simulink model "OswaldE_Proj2_Sim"  (R2024b)
settings: Solver=ode45  StartTime=0.0  StopTime=300  RelTol=1e-3  AbsTol=1e-6
values from neighbouring files (symbols this model uses):
  g0 = 32.17    [OswaldE_Proj2_Code.m]
  gamma_0 = 0    [OswaldE_Proj2_Code.m]
  h_0 = 20000    [OswaldE_Proj2_Code.m]
  K_f = 4*10^-6    (= 4e-06)    [OswaldE_Proj2_Code.m]
  K_L_max = 2.6    [OswaldE_Proj2_Code.m]
  K_mu_p = 0.075    [OswaldE_Proj2_Code.m]
  KL_i = 0.01    [OswaldE_Proj2_Code.m]
  KL_p = 0.5    [OswaldE_Proj2_Code.m]
  KT_i = 0.002    [OswaldE_Proj2_Code.m]
  KT_p = 0.08    [OswaldE_Proj2_Code.m]
  lat_0 = 33.2098 * pi/180    (= 0.579620353929)    [OswaldE_Proj2_Code.m]
  long_0 = -87.5692 * pi/180    (= -1.52837086334)    [OswaldE_Proj2_Code.m]
  mu_max = 30    [OswaldE_Proj2_Code.m]
  omega_L = 2.5    [OswaldE_Proj2_Code.m]
  omega_mu = 1    [OswaldE_Proj2_Code.m]
  omega_t = 2    [OswaldE_Proj2_Code.m]
  sigma_0 = 0    [OswaldE_Proj2_Code.m]
  T_max = 72000    [OswaldE_Proj2_Code.m]
  v_bn_0 = 600    [OswaldE_Proj2_Code.m]
  weight_0 = 200000    [OswaldE_Proj2_Code.m]
libraries: simulink_extras x8, simulink x2
settings Model: Creator=jdlarson1  LastModifiedBy=ethan
settings SolverCC: AlgebraicLoopSolver=TrustRegion
settings DataIOCC: SaveFormat=Array  SignalLoggingSaveFormat=ModelDataLogs  ReturnWorkspaceOutputs=off
settings OptimizationCC: BlockReduction=off  BooleanDataType=off  ReuseModelBlockBuffer=off
settings DebuggingCC: SaveWithParameterizedLinksMsg=none  UnderspecifiedInitializationDetection=Classic  MergeDetectMultiDrivingBlocksExec=none  SignalResolutionControl=TryResolveAllWithWarning  MultiTaskDSMMsg=warning  MultiTaskCondExecSysMsg=none  UnconnectedInputMsg=warning  UnconnectedOutputMsg=warning  UnconnectedLineMsg=warning
settings HardwareCC: TargetUnknown=on
settings ModelReferenceCC: EnableRefExpFcnMdlSchedulingChecks=on  PropagateSignalLabelsOutOfModel=off
settings RTWCC: GPUComputeCapability=3.5  DLArmComputeVersion=19.05
settings GRTTargetCC: CombineOutputUpdateFcns=off  GRTInterface=on

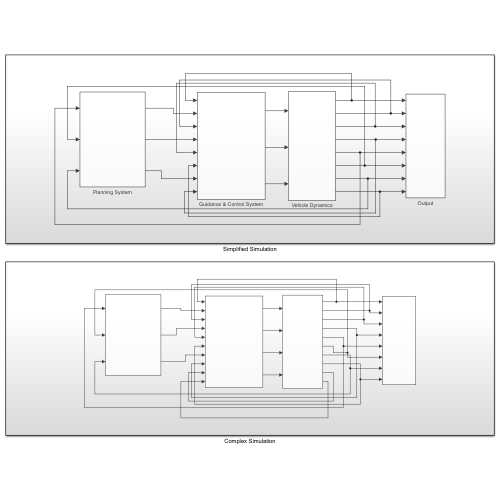
[thumbnail: Simulink's stored preview of the top-level diagram]
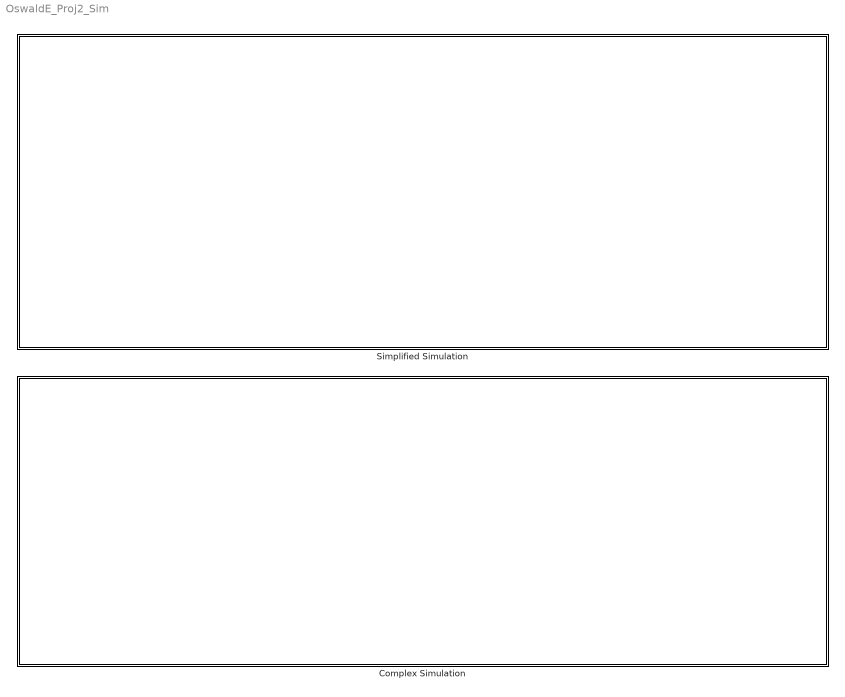
== system OswaldE_Proj2_Sim ==
  Complex Simulation : Subsystem
  Simplified Simulation : Subsystem

== system OswaldE_Proj2_Sim/Complex Simulation ==
  Guidance & Control System1 : Subsystem
  Output1 : Subsystem
  Planning System1 : Subsystem
  Vehicle Dynamics1 : Subsystem
  wires:
  Vehicle Dynamics1/2(" groundspeed ") -> Output1/2(groundspeed), Guidance & Control System1/3(groundspeed)
  Planning System1/2(flight-path_com) -> Guidance & Control System1/4(flight-path_com)
  Vehicle Dynamics1/3(" flight-path ") -> Output1/3(flight-path), Guidance & Control System1/5(flight-path)
  Vehicle Dynamics1/4(" heading ") -> Guidance & Control System1/8(heading), Output1/4(heading)
  Vehicle Dynamics1/7(altitude) -> Planning System1/3(altitude), Output1/7(altitude)
  Vehicle Dynamics1/10(rho) -> Guidance & Control System1/10(rho)
  Guidance & Control System1/3(bank) -> Vehicle Dynamics1/3(bank)
  Vehicle Dynamics1/8(airspeed) -> Guidance & Control System1/6(airspeed), Output1/8(airspeed)
  Vehicle Dynamics1/5(latitude) -> Planning System1/1(latitude), Output1/5(latitude)
  Planning System1/3(heading_com) -> Guidance & Control System1/7(heading_com)
  Vehicle Dynamics1/6(longitude) -> Output1/6(longitude), Planning System1/2(longitude)
  Guidance & Control System1/4(alpha) -> Vehicle Dynamics1/4(alpha)
  Vehicle Dynamics1/1(" mass") -> Guidance & Control System1/1(mass), Output1/1(mass)
  Guidance & Control System1/1(thrust) -> Vehicle Dynamics1/1("thrust ")
  Guidance & Control System1/2(lift) -> Vehicle Dynamics1/2("lift ")
  Planning System1/1(groundspeed_com) -> Guidance & Control System1/2(groundspeed_com)
  Vehicle Dynamics1/9(g) -> Guidance & Control System1/9(g)

== system OswaldE_Proj2_Sim/Simplified Simulation ==
  Guidance & Control System : Subsystem
  Output : Subsystem
  Planning System : Subsystem
  Vehicle Dynamics : Subsystem
  wires:
  Vehicle Dynamics/2(" groundspeed ") -> Guidance & Control System/3(groundspeed), Output/2(groundspeed)
  Vehicle Dynamics/5(latitude) -> Planning System/1(latitude), Output/5(latitude)
  Vehicle Dynamics/7(altitude) -> Planning System/3(altitude), Output/7(altitude)
  Vehicle Dynamics/3(" flight-path ") -> Guidance & Control System/5(flight-path), Output/3(flight-path)
  Planning System/1(groundspeed_com) -> Guidance & Control System/2(groundspeed_com)
  Guidance & Control System/2(lift) -> Vehicle Dynamics/2("lift ")
  Guidance & Control System/1(thrust) -> Vehicle Dynamics/1("thrust ")
  Vehicle Dynamics/1(" mass") -> Output/1(mass), Guidance & Control System/1(mass)
  Vehicle Dynamics/4(" heading ") -> Guidance & Control System/8(heading), Output/4(heading)
  Guidance & Control System/3(bank) -> Vehicle Dynamics/3(bank)
  Vehicle Dynamics/8(airspeed) -> Guidance & Control System/6(airspeed), Output/8(airspeed)
  Vehicle Dynamics/6(longitude) -> Planning System/2(longitude), Output/6(longitude)
  Planning System/3(heading_com) -> Guidance & Control System/7(heading_com)
  Planning System/2(flight-path_com) -> Guidance & Control System/4(flight-path_com)

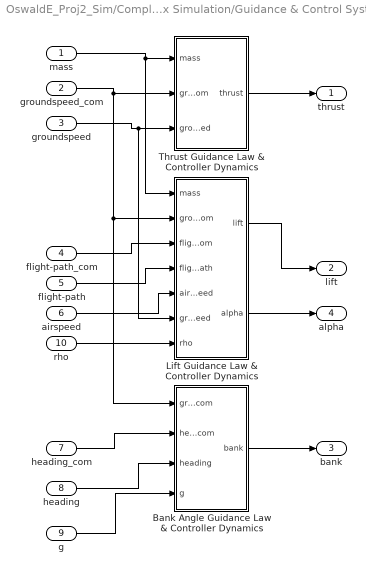
== system OswaldE_Proj2_Sim/Complex Simulation/Guidance & Control System1 ==
  mass : Inport
  groundspeed_com : Inport  Port=2
  groundspeed : Inport  Port=3
  flight-path_com : Inport  Port=4
  flight-path : Inport  Port=5
  airspeed : Inport  Port=6
  heading_com : Inport  Port=7
  heading : Inport  Port=8
  g : Inport  Port=9
  rho : Inport  Port=10
  Bank Angle Guidance Law & Controller Dynamics : Subsystem
  Lift Guidance Law & Controller Dynamics : Subsystem
  Thrust Guidance Law & Controller Dynamics : Subsystem
  thrust : Outport
  lift : Outport  Port=2
  bank : Outport  Port=3
  alpha : Outport  Port=4
  wires:
  mass/1 -> Lift Guidance Law & Controller Dynamics/1(mass), Thrust Guidance Law & Controller Dynamics/1(mass)
  heading_com/1 -> Bank Angle Guidance Law & Controller Dynamics/2(heading_com)
  groundspeed/1 -> Thrust Guidance Law & Controller Dynamics/3(groundspeed), Lift Guidance Law & Controller Dynamics/6(groundspeed)
  groundspeed_com/1 -> Bank Angle Guidance Law & Controller Dynamics/1(groundspeed_com), Lift Guidance Law & Controller Dynamics/2(groundspeed_com), Thrust Guidance Law & Controller Dynamics/2(groundspeed_com)
  heading/1 -> Bank Angle Guidance Law & Controller Dynamics/3(heading)
  flight-path/1 -> Lift Guidance Law & Controller Dynamics/4(flight_path)
  airspeed/1 -> Lift Guidance Law & Controller Dynamics/5(airspeed)
  Thrust Guidance Law & Controller Dynamics/1(thrust) -> thrust/1
  Lift Guidance Law & Controller Dynamics/1(lift) -> lift/1
  Bank Angle Guidance Law & Controller Dynamics/1(bank) -> bank/1
  flight-path_com/1 -> Lift Guidance Law & Controller Dynamics/3(flight_path_com)
  g/1 -> Bank Angle Guidance Law & Controller Dynamics/4(g)
  Lift Guidance Law & Controller Dynamics/2(alpha) -> alpha/1
  rho/1 -> Lift Guidance Law & Controller Dynamics/7(rho)

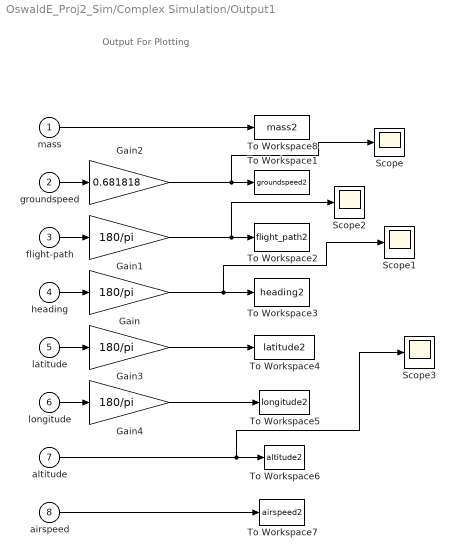
== system OswaldE_Proj2_Sim/Complex Simulation/Output1 ==
  note: Output For Plotting
  mass : Inport
  groundspeed : Inport  Port=2
  flight-path : Inport  Port=3
  heading : Inport  Port=4
  latitude : Inport  Port=5
  longitude : Inport  Port=6
  altitude : Inport  Port=7
  airspeed : Inport  Port=8
  Gain{,1,3..4} (4 alike) : Gain  Gain=180/pi
  Gain2 : Gain  Gain=0.681818
  Scope{,1..3} (4 alike) : Scope
  To Workspace1 : ToWorkspace  VariableName=groundspeed2
  To Workspace2 : ToWorkspace  VariableName=flight_path2
  To Workspace3 : ToWorkspace  VariableName=heading2
  To Workspace4 : ToWorkspace  VariableName=latitude2
  To Workspace5 : ToWorkspace  VariableName=longitude2
  To Workspace6 : ToWorkspace  VariableName=altitude2
  To Workspace7 : ToWorkspace  VariableName=airspeed2
  To Workspace8 : ToWorkspace  VariableName=mass2
  wires:
  latitude/1 -> Gain3/1
  groundspeed/1 -> Gain2/1
  flight-path/1 -> Gain1/1
  heading/1 -> Gain/1
  longitude/1 -> Gain4/1
  altitude/1 -> Scope3/1, To Workspace6/1
  Gain2/1 -> Scope/1, To Workspace1/1
  Gain1/1 -> Scope2/1, To Workspace2/1
  Gain/1 -> Scope1/1, To Workspace3/1
  airspeed/1 -> To Workspace7/1
  mass/1 -> To Workspace8/1
  Gain3/1 -> To Workspace4/1
  Gain4/1 -> To Workspace5/1

== system OswaldE_Proj2_Sim/Complex Simulation/Planning System1 ==
  latitude : Inport
  longitude : Inport  Port=2
  altitude : Inport  Port=3
  CD1 : Gain  Gain=180/pi  SaturateOnIntegerOverflow=on
  CD7 : Gain  Gain=180/pi  SaturateOnIntegerOverflow=on
  CD8 : Gain  Gain=0.681818  SaturateOnIntegerOverflow=on
  Command System : MATLAB Function  TreatAsAtomicUnit=on
  To Workspace10 : ToWorkspace  VariableName=heading_com2
  To Workspace5 : ToWorkspace  VariableName=groundspeed_com2
  To Workspace7 : ToWorkspace  VariableName=flight_path_com2
  groundspeed_com : Outport
  flight-path_com : Outport  Port=2
  heading_com : Outport  Port=3
  wires:
  latitude/1 -> Command System/1(latitude)
  longitude/1 -> Command System/2(longitude)
  altitude/1 -> Command System/3(altitude)
  Command System/1(groundspeed_com) -> CD8/1, groundspeed_com/1
  Command System/2(flight_path_com) -> CD7/1, flight-path_com/1
  Command System/3(heading_com) -> CD1/1, heading_com/1
  CD8/1 -> To Workspace5/1
  CD7/1 -> To Workspace7/1
  CD1/1 -> To Workspace10/1

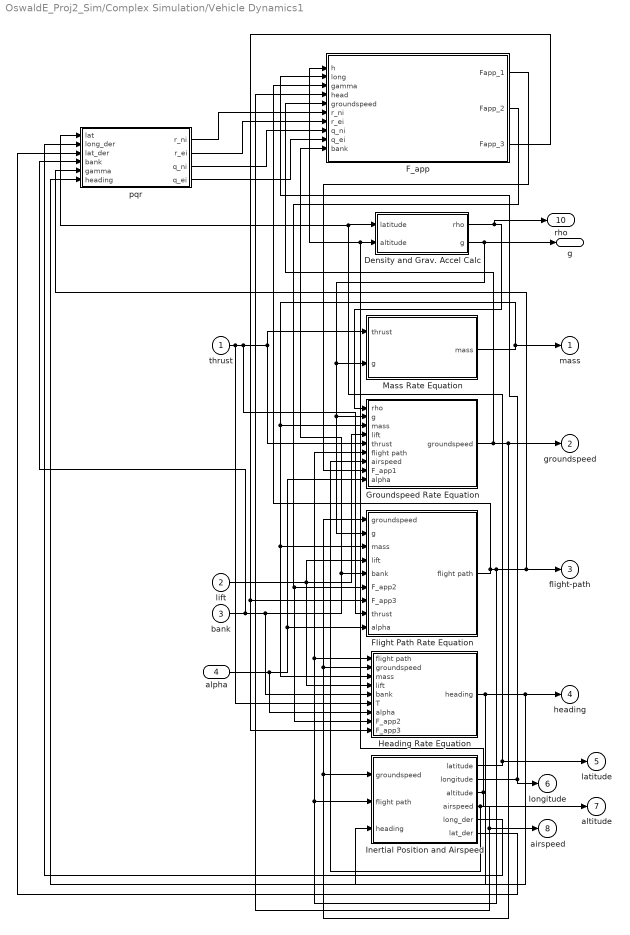
== system OswaldE_Proj2_Sim/Complex Simulation/Vehicle Dynamics1 ==
  "thrust " : Inport
  "lift " : Inport  Port=2
  bank : Inport  Port=3
  alpha : Inport  Port=4
  Density and Grav. Accel Calc : Subsystem
  F_app : Subsystem
  Flight Path Rate Equation : Subsystem
  Groundspeed Rate Equation : Subsystem
  Heading Rate Equation : Subsystem
  Inertial Position and Airspeed : Subsystem
  Mass Rate Equation : Subsystem
  pqr : Subsystem
  " mass" : Outport
  " groundspeed " : Outport  Port=2
  " flight-path " : Outport  Port=3
  " heading " : Outport  Port=4
  latitude : Outport  Port=5
  longitude : Outport  Port=6
  altitude : Outport  Port=7
  airspeed : Outport  Port=8
  g : Outport  Port=9
  rho : Outport  Port=10
  wires:
  bank/1 -> pqr/4(bank), F_app/10(bank), Flight Path Rate Equation/5(bank), Heading Rate Equation/5(bank)
  "lift "/1 -> Heading Rate Equation/4("lift "), Flight Path Rate Equation/4("lift "), Groundspeed Rate Equation/4(lift)
  "thrust "/1 -> Heading Rate Equation/6(T), Flight Path Rate Equation/8(thrust), Groundspeed Rate Equation/5(thrust), Mass Rate Equation/1(thrust)
  Heading Rate Equation/1(heading) -> Inertial Position and Airspeed/3(heading), " heading "/1, pqr/6(heading)
  Flight Path Rate Equation/1(flight path) -> F_app/3(gamma), Groundspeed Rate Equation/6(flight path), Heading Rate Equation/1(flight path), Inertial Position and Airspeed/2("flight path "), pqr/5(gamma), " flight-path "/1
  Groundspeed Rate Equation/1(groundspeed) -> F_app/5(groundspeed), Flight Path Rate Equation/1(groundspeed), Heading Rate Equation/2(groundspeed), Inertial Position and Airspeed/1(groundspeed), " groundspeed "/1
  Inertial Position and Airspeed/2(longitude) -> longitude/1, F_app/2(long)
  Inertial Position and Airspeed/4(airspeed) -> F_app/4(head), airspeed/1, Groundspeed Rate Equation/7(airspeed)
  Inertial Position and Airspeed/1(latitude) -> pqr/1(lat), Density and Grav. Accel Calc/1(latitude), latitude/1
  Inertial Position and Airspeed/3(altitude) -> altitude/1, F_app/1(h), Density and Grav. Accel Calc/2(altitude)
  Mass Rate Equation/1("mass ") -> " mass"/1, Heading Rate Equation/3(mass), Flight Path Rate Equation/3(mass), Groundspeed Rate Equation/3(mass)
  Density and Grav. Accel Calc/1(rho) -> rho/1, Groundspeed Rate Equation/1(rho)
  Density and Grav. Accel Calc/2(g) -> g/1, Flight Path Rate Equation/2(g), Groundspeed Rate Equation/2(g), Mass Rate Equation/2(g)
  pqr/1(r_ni) -> F_app/6(r_ni)
  pqr/2(r_ei) -> F_app/7(r_ei)
  pqr/3(q_ni) -> F_app/8(q_ni)
  pqr/4(q_ei) -> F_app/9(q_ei)
  Inertial Position and Airspeed/5(long_der) -> pqr/2(long_der)
  Inertial Position and Airspeed/6(lat_der) -> pqr/3(lat_der)
  F_app/1(Fapp_1) -> Groundspeed Rate Equation/8(F_app1)
  F_app/2(Fapp_2) -> Heading Rate Equation/8(F_app2), Flight Path Rate Equation/6(F_app2)
  F_app/3(Fapp_3) -> Heading Rate Equation/9(F_app3), Flight Path Rate Equation/7(F_app3)
  alpha/1 -> Heading Rate Equation/7(alpha), Groundspeed Rate Equation/9(alpha), Flight Path Rate Equation/9(alpha)

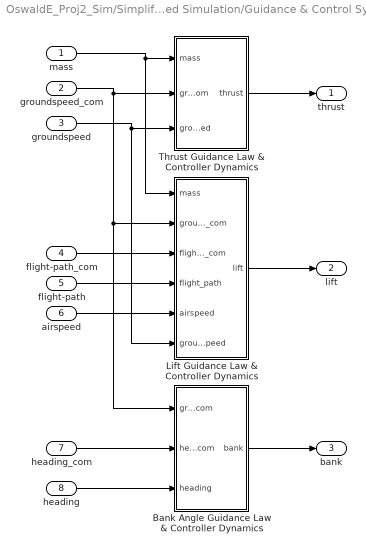
== system OswaldE_Proj2_Sim/Simplified Simulation/Guidance & Control System ==
  mass : Inport
  groundspeed_com : Inport  Port=2
  groundspeed : Inport  Port=3
  flight-path_com : Inport  Port=4
  flight-path : Inport  Port=5
  airspeed : Inport  Port=6
  heading_com : Inport  Port=7
  heading : Inport  Port=8
  Bank Angle Guidance Law & Controller Dynamics : Subsystem
  Lift Guidance Law & Controller Dynamics : Subsystem
  Thrust Guidance Law & Controller Dynamics : Subsystem
  thrust : Outport
  lift : Outport  Port=2
  bank : Outport  Port=3
  wires:
  mass/1 -> Lift Guidance Law & Controller Dynamics/1(mass), Thrust Guidance Law & Controller Dynamics/1(mass)
  heading_com/1 -> Bank Angle Guidance Law & Controller Dynamics/2(heading_com)
  groundspeed/1 -> Thrust Guidance Law & Controller Dynamics/3(groundspeed), Lift Guidance Law & Controller Dynamics/6(groundspeed)
  groundspeed_com/1 -> Lift Guidance Law & Controller Dynamics/2(groundspeed_com), Bank Angle Guidance Law & Controller Dynamics/1(groundspeed_com), Thrust Guidance Law & Controller Dynamics/2(groundspeed_com)
  heading/1 -> Bank Angle Guidance Law & Controller Dynamics/3(heading)
  flight-path/1 -> Lift Guidance Law & Controller Dynamics/4(flight_path)
  airspeed/1 -> Lift Guidance Law & Controller Dynamics/5(airspeed)
  Thrust Guidance Law & Controller Dynamics/1(thrust) -> thrust/1
  Lift Guidance Law & Controller Dynamics/1(lift) -> lift/1
  Bank Angle Guidance Law & Controller Dynamics/1(bank) -> bank/1
  flight-path_com/1 -> Lift Guidance Law & Controller Dynamics/3(flight_path_com)

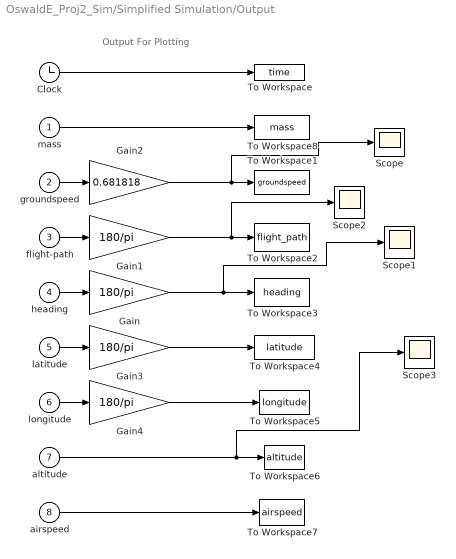
== system OswaldE_Proj2_Sim/Simplified Simulation/Output ==
  note: Output For Plotting
  mass : Inport
  groundspeed : Inport  Port=2
  flight-path : Inport  Port=3
  heading : Inport  Port=4
  latitude : Inport  Port=5
  longitude : Inport  Port=6
  altitude : Inport  Port=7
  airspeed : Inport  Port=8
  Clock : Clock
  Gain{,1,3..4} (4 alike) : Gain  Gain=180/pi
  Gain2 : Gain  Gain=0.681818
  Scope{,1..3} (4 alike) : Scope
  To Workspace : ToWorkspace  VariableName=time
  To Workspace1 : ToWorkspace  VariableName=groundspeed
  To Workspace2 : ToWorkspace  VariableName=flight_path
  To Workspace3 : ToWorkspace  VariableName=heading
  To Workspace4 : ToWorkspace  VariableName=latitude
  To Workspace5 : ToWorkspace  VariableName=longitude
  To Workspace6 : ToWorkspace  VariableName=altitude
  To Workspace7 : ToWorkspace  VariableName=airspeed
  To Workspace8 : ToWorkspace  VariableName=mass
  wires:
  Clock/1 -> To Workspace/1
  latitude/1 -> Gain3/1
  groundspeed/1 -> Gain2/1
  flight-path/1 -> Gain1/1
  heading/1 -> Gain/1
  longitude/1 -> Gain4/1
  altitude/1 -> Scope3/1, To Workspace6/1
  Gain2/1 -> Scope/1, To Workspace1/1
  Gain1/1 -> Scope2/1, To Workspace2/1
  Gain/1 -> Scope1/1, To Workspace3/1
  airspeed/1 -> To Workspace7/1
  mass/1 -> To Workspace8/1
  Gain3/1 -> To Workspace4/1
  Gain4/1 -> To Workspace5/1

== system OswaldE_Proj2_Sim/Simplified Simulation/Planning System ==
  latitude : Inport
  longitude : Inport  Port=2
  altitude : Inport  Port=3
  CD1 : Gain  Gain=180/pi  SaturateOnIntegerOverflow=on
  CD7 : Gain  Gain=180/pi  SaturateOnIntegerOverflow=on
  CD8 : Gain  Gain=0.681818  SaturateOnIntegerOverflow=on
  Command System : MATLAB Function  TreatAsAtomicUnit=on
  To Workspace10 : ToWorkspace  VariableName=heading_com
  To Workspace5 : ToWorkspace  VariableName=groundspeed_com
  To Workspace7 : ToWorkspace  VariableName=flight_path_com
  groundspeed_com : Outport
  flight-path_com : Outport  Port=2
  heading_com : Outport  Port=3
  wires:
  latitude/1 -> Command System/1(latitude)
  longitude/1 -> Command System/2(longitude)
  altitude/1 -> Command System/3(altitude)
  Command System/1(groundspeed_com) -> CD8/1, groundspeed_com/1
  Command System/2(flight_path_com) -> CD7/1, flight-path_com/1
  Command System/3(heading_com) -> CD1/1, heading_com/1
  CD8/1 -> To Workspace5/1
  CD7/1 -> To Workspace7/1
  CD1/1 -> To Workspace10/1

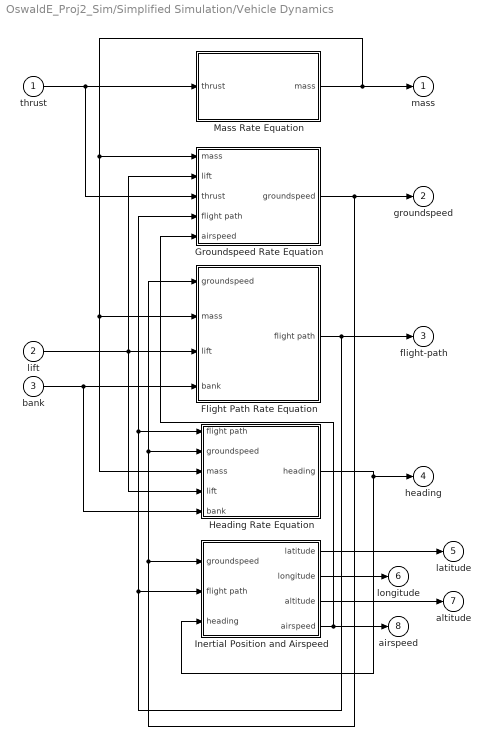
== system OswaldE_Proj2_Sim/Simplified Simulation/Vehicle Dynamics ==
  "thrust " : Inport
  "lift " : Inport  Port=2
  bank : Inport  Port=3
  Flight Path Rate Equation : Subsystem
  Groundspeed Rate Equation : Subsystem
  Heading Rate Equation : Subsystem
  Inertial Position and Airspeed : Subsystem
  Mass Rate Equation : Subsystem
  " mass" : Outport
  " groundspeed " : Outport  Port=2
  " flight-path " : Outport  Port=3
  " heading " : Outport  Port=4
  latitude : Outport  Port=5
  longitude : Outport  Port=6
  altitude : Outport  Port=7
  airspeed : Outport  Port=8
  wires:
  bank/1 -> Heading Rate Equation/5(bank), Flight Path Rate Equation/4(bank)
  "lift "/1 -> Heading Rate Equation/4("lift "), Flight Path Rate Equation/3("lift "), Groundspeed Rate Equation/2(lift)
  "thrust "/1 -> Groundspeed Rate Equation/3(thrust), Mass Rate Equation/1(thrust)
  Heading Rate Equation/1(heading) -> Inertial Position and Airspeed/3(heading), " heading "/1
  Flight Path Rate Equation/1(flight path) -> Groundspeed Rate Equation/4(flight path), Heading Rate Equation/1(flight path), Inertial Position and Airspeed/2("flight path "), " flight-path "/1
  Groundspeed Rate Equation/1(groundspeed) -> Flight Path Rate Equation/1(groundspeed), Heading Rate Equation/2(groundspeed), Inertial Position and Airspeed/1(groundspeed), " groundspeed "/1
  Inertial Position and Airspeed/2(longitude) -> longitude/1
  Inertial Position and Airspeed/4(airspeed) -> Groundspeed Rate Equation/5(airspeed), airspeed/1
  Inertial Position and Airspeed/1(latitude) -> latitude/1
  Inertial Position and Airspeed/3(altitude) -> altitude/1
  Mass Rate Equation/1("mass ") -> " mass"/1, Heading Rate Equation/3(mass), Flight Path Rate Equation/2(mass), Groundspeed Rate Equation/1(mass)

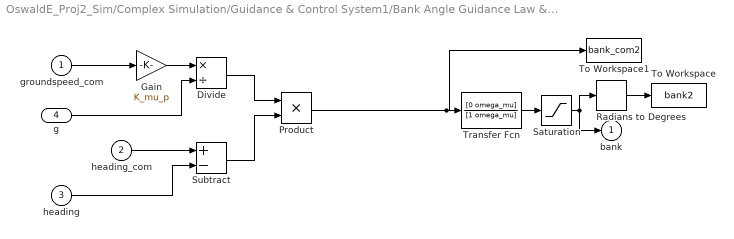
== system OswaldE_Proj2_Sim/Complex Simulation/Guidance & Control System1/Bank Angle Guidance Law & Controller Dynamics ==
  groundspeed_com : Inport
  heading_com : Inport  Port=2
  heading : Inport  Port=3
  g : Inport  Port=4
  Divide : Product  Inputs=*/
  Gain : Gain  Gain=K_mu_p
  Product : Product
  Radians to Degrees : simulink_extras/Transformations/Radians to Degrees
  Saturation : Saturate  UpperLimit=mu_max*pi/180  LowerLimit=-mu_max*pi/180
  Subtract : Sum  Inputs=+-
  To Workspace : ToWorkspace  VariableName=bank2
  To Workspace1 : ToWorkspace  VariableName=bank_com2
  Transfer Fcn : TransferFcn  Numerator=[0 omega_mu]  Denominator=[1 omega_mu]
  bank : Outport
  wires:
  groundspeed_com/1 -> Gain/1
  Gain/1 -> Divide/1
  g/1 -> Divide/2
  heading_com/1 -> Subtract/1
  heading/1 -> Subtract/2
  Divide/1 -> Product/1
  Subtract/1 -> Product/2
  Product/1 -> To Workspace1/1, Transfer Fcn/1
  Transfer Fcn/1 -> Saturation/1
  Saturation/1 -> bank/1, Radians to Degrees/1
  Radians to Degrees/1 -> To Workspace/1

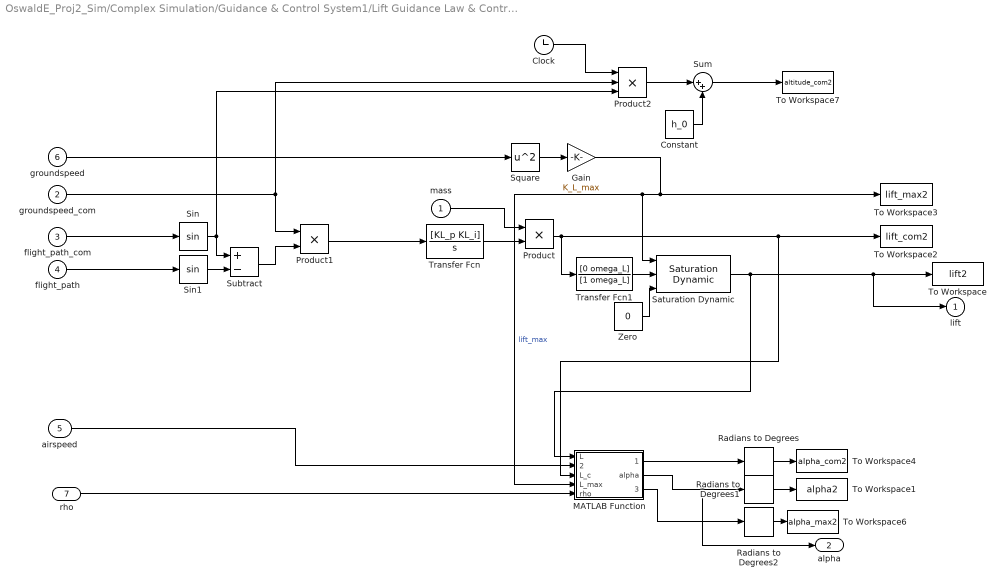
== system OswaldE_Proj2_Sim/Complex Simulation/Guidance & Control System1/Lift Guidance Law & Controller Dynamics ==
  mass : Inport
  groundspeed_com : Inport  Port=2
  flight_path_com : Inport  Port=3
  flight_path : Inport  Port=4
  airspeed : Inport  Port=5
  groundspeed : Inport  Port=6
  rho : Inport  Port=7
  Clock : Clock
  Constant : Constant  Value=h_0
  Gain : Gain  Gain=K_L_max
  MATLAB Function : MATLAB Function  TreatAsAtomicUnit=on
  Product : Product
  Product1 : Product
  Product2 : Product  Inputs=3
  Radians to Degrees : simulink_extras/Transformations/Radians to Degrees
  Radians to Degrees1 : simulink_extras/Transformations/Radians to Degrees
  Radians to Degrees2 : simulink_extras/Transformations/Radians to Degrees
  Saturation Dynamic : simulink/Discontinuities/Saturation Dynamic  OutMin=[]  OutMax=[]  OutDataTypeStr=Inherit: Same as second input  OutDataType=fixdt(1, 16)  OutScaling=2^-10  DoSatur=off
  Sin : Trigonometry
  Sin1 : Trigonometry
  Square : Math  Operator=square
  Subtract : Sum  Inputs=+-
  Sum : Sum  Inputs=|++
  To Workspace : ToWorkspace  VariableName=lift2
  To Workspace1 : ToWorkspace  VariableName=alpha2
  To Workspace2 : ToWorkspace  VariableName=lift_com2
  To Workspace3 : ToWorkspace  VariableName=lift_max2
  To Workspace4 : ToWorkspace  VariableName=alpha_com2
  To Workspace6 : ToWorkspace  VariableName=alpha_max2
  To Workspace7 : ToWorkspace  VariableName=altitude_com2
  Transfer Fcn : TransferFcn  Numerator=[KL_p KL_i]  Denominator=[1 0]
  Transfer Fcn1 : TransferFcn  Numerator=[0 omega_L]  Denominator=[1 omega_L]
  Zero : Constant  Value=0  OutDataTypeStr=Inherit: Inherit via back propagation
  lift : Outport
  alpha : Outport  Port=2
  wires:
  Transfer Fcn/1 -> Product/2
  mass/1 -> Product/1
  flight_path_com/1 -> Sin/1
  Sin/1 -> Subtract/1, Product2/3
  flight_path/1 -> Sin1/1
  Sin1/1 -> Subtract/2
  Subtract/1 -> Product1/2
  groundspeed_com/1 -> Product2/2, Product1/1
  Product1/1 -> Transfer Fcn/1
  Product/1 -> Transfer Fcn1/1, MATLAB Function/3(L_c), To Workspace2/1
  groundspeed/1 -> Square/1
  Square/1 -> Gain/1
  Gain/1 -> MATLAB Function/4(L_max), Saturation Dynamic/1, To Workspace3/1  "lift_max"
  airspeed/1 -> MATLAB Function/2(airspeed)
  MATLAB Function/2(alpha) -> Radians to Degrees1/1, alpha/1
  Transfer Fcn1/1 -> Saturation Dynamic/2
  Saturation Dynamic/1 -> MATLAB Function/1(L), lift/1, To Workspace/1
  Zero/1 -> Saturation Dynamic/3
  Clock/1 -> Product2/1
  Product2/1 -> Sum/1
  Constant/1 -> Sum/2
  Sum/1 -> To Workspace7/1
  rho/1 -> MATLAB Function/5(rho)
  Radians to Degrees/1 -> To Workspace4/1
  MATLAB Function/1(alpha_c) -> Radians to Degrees/1
  Radians to Degrees1/1 -> To Workspace1/1
  MATLAB Function/3(alpha_max) -> Radians to Degrees2/1
  Radians to Degrees2/1 -> To Workspace6/1

== system OswaldE_Proj2_Sim/Complex Simulation/Guidance & Control System1/Thrust Guidance Law & Controller Dynamics ==
  mass : Inport
  groundspeed_com : Inport  Port=2
  groundspeed : Inport  Port=3
  Product : Product
  Saturation : Saturate  UpperLimit=T_max  LowerLimit=0
  Subtract : Sum  Inputs=+-
  To Workspace : ToWorkspace  VariableName=thrust2
  To Workspace1 : ToWorkspace  VariableName=thrust_com2
  Transfer Fcn : TransferFcn  Numerator=[KT_p KT_i]  Denominator=[1 0]
  Transfer Fcn1 : TransferFcn  Numerator=[0 omega_t]  Denominator=[1 omega_t]
  thrust : Outport
  wires:
  Transfer Fcn/1 -> Product/2
  mass/1 -> Product/1
  groundspeed_com/1 -> Subtract/1
  groundspeed/1 -> Subtract/2
  Subtract/1 -> Transfer Fcn/1
  Product/1 -> To Workspace1/1, Transfer Fcn1/1
  Transfer Fcn1/1 -> Saturation/1
  Saturation/1 -> thrust/1, To Workspace/1

== system OswaldE_Proj2_Sim/Complex Simulation/Vehicle Dynamics1/Density and Grav. Accel Calc ==
  latitude : Inport
  altitude : Inport  Port=2
  MATLAB Function : MATLAB Function  TreatAsAtomicUnit=on
  rho : Outport
  g : Outport  Port=2
  wires:
  altitude/1 -> MATLAB Function/1(h)
  latitude/1 -> MATLAB Function/2(lat)
  MATLAB Function/1(rho) -> rho/1
  MATLAB Function/2(g) -> g/1

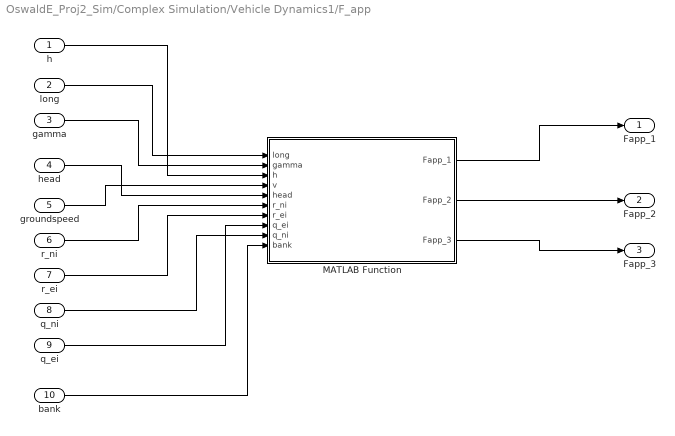
== system OswaldE_Proj2_Sim/Complex Simulation/Vehicle Dynamics1/F_app ==
  h : Inport
  long : Inport  Port=2
  gamma : Inport  Port=3
  head : Inport  Port=4
  groundspeed : Inport  Port=5
  r_ni : Inport  Port=6
  r_ei : Inport  Port=7
  q_ni : Inport  Port=8
  q_ei : Inport  Port=9
  bank : Inport  Port=10
  MATLAB Function : MATLAB Function  TreatAsAtomicUnit=on
  Fapp_1 : Outport
  Fapp_2 : Outport  Port=2
  Fapp_3 : Outport  Port=3
  wires:
  h/1 -> MATLAB Function/3(h)
  long/1 -> MATLAB Function/1(long)
  gamma/1 -> MATLAB Function/2(gamma)
  head/1 -> MATLAB Function/5(head)
  groundspeed/1 -> MATLAB Function/4(v)
  r_ni/1 -> MATLAB Function/6(r_ni)
  r_ei/1 -> MATLAB Function/7(r_ei)
  q_ni/1 -> MATLAB Function/9(q_ni)
  q_ei/1 -> MATLAB Function/8(q_ei)
  MATLAB Function/1(Fapp_1) -> Fapp_1/1
  MATLAB Function/2(Fapp_2) -> Fapp_2/1
  MATLAB Function/3(Fapp_3) -> Fapp_3/1
  bank/1 -> MATLAB Function/10(bank)

== system OswaldE_Proj2_Sim/Complex Simulation/Vehicle Dynamics1/Flight Path Rate Equation ==
  groundspeed : Inport
  g : Inport  Port=2
  mass : Inport  Port=3
  "lift " : Inport  Port=4
  bank : Inport  Port=5
  F_app2 : Inport  Port=6
  F_app3 : Inport  Port=7
  thrust : Inport  Port=8
  alpha : Inport  Port=9
  Integrator : Integrator  InitialCondition=gamma_0
  MATLAB Function : MATLAB Function  TreatAsAtomicUnit=on
  flight path : Outport
  wires:
  groundspeed/1 -> MATLAB Function/2(v)
  mass/1 -> MATLAB Function/5(m)
  "lift "/1 -> MATLAB Function/1(L)
  bank/1 -> MATLAB Function/3(mu)
  MATLAB Function/1(gamma_der) -> Integrator/1
  Integrator/1 -> MATLAB Function/4(gamma), flight path/1
  g/1 -> MATLAB Function/6(g)
  F_app2/1 -> MATLAB Function/7(F_app2)
  F_app3/1 -> MATLAB Function/8(F_app3)
  thrust/1 -> MATLAB Function/10(T)
  alpha/1 -> MATLAB Function/9(alpha)

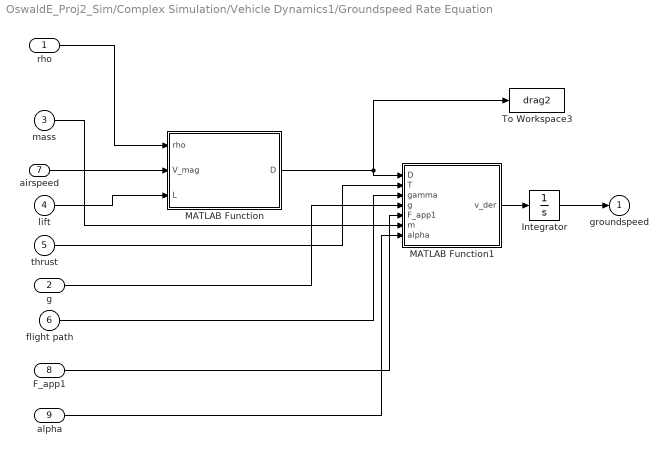
== system OswaldE_Proj2_Sim/Complex Simulation/Vehicle Dynamics1/Groundspeed Rate Equation ==
  rho : Inport
  g : Inport  Port=2
  mass : Inport  Port=3
  lift : Inport  Port=4
  thrust : Inport  Port=5
  flight path : Inport  Port=6
  airspeed : Inport  Port=7
  F_app1 : Inport  Port=8
  alpha : Inport  Port=9
  Integrator : Integrator  InitialCondition=v_bn_0
  MATLAB Function : MATLAB Function  TreatAsAtomicUnit=on
  MATLAB Function1 : MATLAB Function  TreatAsAtomicUnit=on
  To Workspace3 : ToWorkspace  VariableName=drag2
  groundspeed : Outport
  wires:
  airspeed/1 -> MATLAB Function/2(V_mag)
  lift/1 -> MATLAB Function/3(L)
  Integrator/1 -> groundspeed/1
  rho/1 -> MATLAB Function/1(rho)
  MATLAB Function/1(D) -> To Workspace3/1, MATLAB Function1/1(D)
  thrust/1 -> MATLAB Function1/2(T)
  mass/1 -> MATLAB Function1/6(m)
  flight path/1 -> MATLAB Function1/3(gamma)
  MATLAB Function1/1(v_der) -> Integrator/1
  g/1 -> MATLAB Function1/4(g)
  F_app1/1 -> MATLAB Function1/5(F_app1)
  alpha/1 -> MATLAB Function1/7(alpha)

== system OswaldE_Proj2_Sim/Complex Simulation/Vehicle Dynamics1/Heading Rate Equation ==
  flight path : Inport
  groundspeed : Inport  Port=2
  mass : Inport  Port=3
  "lift " : Inport  Port=4
  bank : Inport  Port=5
  T : Inport  Port=6
  alpha : Inport  Port=7
  F_app2 : Inport  Port=8
  F_app3 : Inport  Port=9
  Integrator : Integrator  InitialCondition=sigma_0
  MATLAB Function : MATLAB Function  TreatAsAtomicUnit=on
  heading : Outport
  wires:
  "lift "/1 -> MATLAB Function/1(L)
  bank/1 -> MATLAB Function/3(bank)
  mass/1 -> MATLAB Function/2(m)
  groundspeed/1 -> MATLAB Function/4(v)
  flight path/1 -> MATLAB Function/5(gamma)
  MATLAB Function/1(head_der) -> Integrator/1
  Integrator/1 -> heading/1
  T/1 -> MATLAB Function/6(T)
  alpha/1 -> MATLAB Function/7(alpha)
  F_app2/1 -> MATLAB Function/8(F_app2)
  F_app3/1 -> MATLAB Function/9(F_app3)

== system OswaldE_Proj2_Sim/Complex Simulation/Vehicle Dynamics1/Inertial Position and Airspeed ==
  groundspeed : Inport
  "flight path " : Inport  Port=2
  heading : Inport  Port=3
  Integrator : Integrator  InitialCondition=lat_0
  Integrator1 : Integrator  InitialCondition=long_0
  Integrator2 : Integrator  InitialCondition=h_0
  MATLAB Function : MATLAB Function  TreatAsAtomicUnit=on
  latitude : Outport
  longitude : Outport  Port=2
  altitude : Outport  Port=3
  airspeed : Outport  Port=4
  long_der : Outport  Port=5
  lat_der : Outport  Port=6
  wires:
  MATLAB Function/1(lat_der) -> lat_der/1, Integrator/1
  Integrator/1 -> MATLAB Function/4(lat), latitude/1
  MATLAB Function/2(long_der) -> long_der/1, Integrator1/1
  Integrator1/1 -> longitude/1
  "flight path "/1 -> MATLAB Function/3(gamma)
  heading/1 -> MATLAB Function/2(head)
  groundspeed/1 -> MATLAB Function/1(v)
  MATLAB Function/3(h_der) -> Integrator2/1
  Integrator2/1 -> MATLAB Function/5(h), altitude/1
  MATLAB Function/4(windspeed) -> airspeed/1

== system OswaldE_Proj2_Sim/Complex Simulation/Vehicle Dynamics1/Mass Rate Equation ==
  thrust : Inport
  g : Inport  Port=2
  Gain : Gain  Gain=-K_f
  Integrator : Integrator  InitialCondition=weight_0/g0
  Product : Product
  To Workspace2 : ToWorkspace  VariableName=weight2
  "mass " : Outport
  wires:
  thrust/1 -> Gain/1
  Product/1 -> To Workspace2/1
  Gain/1 -> Integrator/1
  Integrator/1 -> Product/2, "mass "/1
  g/1 -> Product/1

== system OswaldE_Proj2_Sim/Complex Simulation/Vehicle Dynamics1/pqr ==
  lat : Inport
  long_der : Inport  Port=2
  lat_der : Inport  Port=3
  bank : Inport  Port=4
  gamma : Inport  Port=5
  heading : Inport  Port=6
  MATLAB Function : MATLAB Function  TreatAsAtomicUnit=on
  r_ni : Outport
  r_ei : Outport  Port=2
  q_ni : Outport  Port=3
  q_ei : Outport  Port=4
  wires:
  MATLAB Function/4(q_ei) -> q_ei/1
  MATLAB Function/3(q_ni) -> q_ni/1
  MATLAB Function/2(r_ei) -> r_ei/1
  MATLAB Function/1(r_ni) -> r_ni/1
  gamma/1 -> MATLAB Function/4(gamma)
  bank/1 -> MATLAB Function/5(bank)
  heading/1 -> MATLAB Function/6(head)
  lat/1 -> MATLAB Function/1(lat)
  long_der/1 -> MATLAB Function/2(long_der)
  lat_der/1 -> MATLAB Function/3(lat_der)

== system OswaldE_Proj2_Sim/Simplified Simulation/Guidance & Control System/Bank Angle Guidance Law & Controller Dynamics ==
  groundspeed_com : Inport
  heading_com : Inport  Port=2
  heading : Inport  Port=3
  Divide : Product  Inputs=*/
  Gain : Gain  Gain=K_mu_p
  Mass1 : Constant  Value=g0
  Product : Product
  Radians to Degrees : simulink_extras/Transformations/Radians to Degrees
  Saturation : Saturate  UpperLimit=mu_max*pi/180  LowerLimit=-mu_max*pi/180
  Subtract : Sum  Inputs=+-
  To Workspace : ToWorkspace  VariableName=bank
  To Workspace1 : ToWorkspace  VariableName=bank_com
  Transfer Fcn : TransferFcn  Numerator=[0 omega_mu]  Denominator=[1 omega_mu]
  bank : Outport
  wires:
  groundspeed_com/1 -> Gain/1
  Gain/1 -> Divide/1
  Mass1/1 -> Divide/2
  heading_com/1 -> Subtract/1
  heading/1 -> Subtract/2
  Divide/1 -> Product/1
  Subtract/1 -> Product/2
  Product/1 -> To Workspace1/1, Transfer Fcn/1
  Transfer Fcn/1 -> Saturation/1
  Saturation/1 -> bank/1, Radians to Degrees/1
  Radians to Degrees/1 -> To Workspace/1

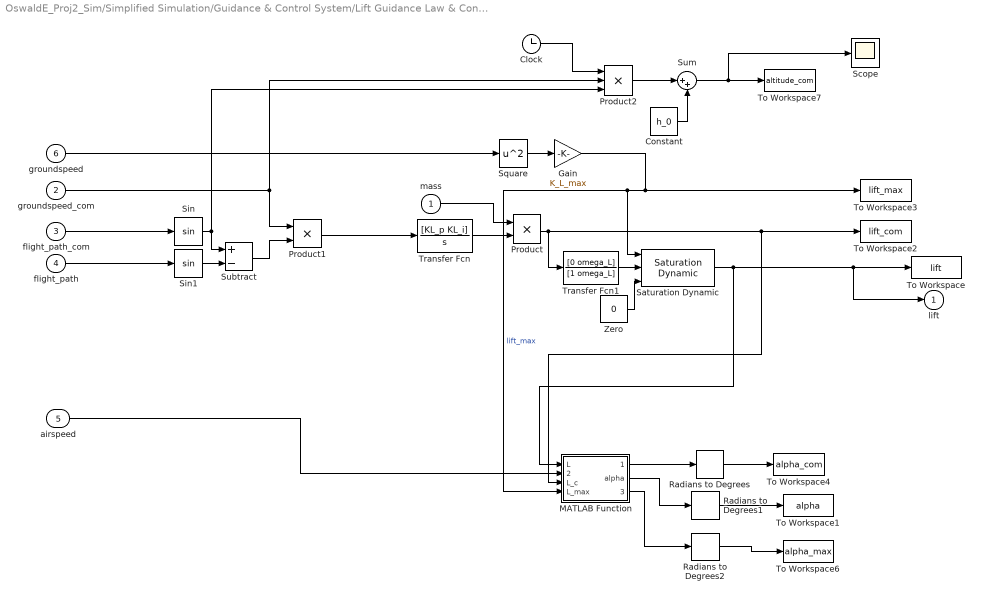
== system OswaldE_Proj2_Sim/Simplified Simulation/Guidance & Control System/Lift Guidance Law & Controller Dynamics ==
  mass : Inport
  groundspeed_com : Inport  Port=2
  flight_path_com : Inport  Port=3
  flight_path : Inport  Port=4
  airspeed : Inport  Port=5
  groundspeed : Inport  Port=6
  Clock : Clock
  Constant : Constant  Value=h_0
  Gain : Gain  Gain=K_L_max
  MATLAB Function : MATLAB Function  TreatAsAtomicUnit=on
  Product : Product
  Product1 : Product
  Product2 : Product  Inputs=3
  Radians to Degrees : simulink_extras/Transformations/Radians to Degrees
  Radians to Degrees1 : simulink_extras/Transformations/Radians to Degrees
  Radians to Degrees2 : simulink_extras/Transformations/Radians to Degrees
  Saturation Dynamic : simulink/Discontinuities/Saturation Dynamic  OutMin=[]  OutMax=[]  OutDataTypeStr=Inherit: Same as second input  OutDataType=fixdt(1, 16)  OutScaling=2^-10  DoSatur=off
  Scope : Scope
  Sin : Trigonometry
  Sin1 : Trigonometry
  Square : Math  Operator=square
  Subtract : Sum  Inputs=+-
  Sum : Sum  Inputs=|++
  To Workspace : ToWorkspace  VariableName=lift
  To Workspace1 : ToWorkspace  VariableName=alpha
  To Workspace2 : ToWorkspace  VariableName=lift_com
  To Workspace3 : ToWorkspace  VariableName=lift_max
  To Workspace4 : ToWorkspace  VariableName=alpha_com
  To Workspace6 : ToWorkspace  VariableName=alpha_max
  To Workspace7 : ToWorkspace  VariableName=altitude_com
  Transfer Fcn : TransferFcn  Numerator=[KL_p KL_i]  Denominator=[1 0]
  Transfer Fcn1 : TransferFcn  Numerator=[0 omega_L]  Denominator=[1 omega_L]
  Zero : Constant  Value=0  OutDataTypeStr=Inherit: Inherit via back propagation
  lift : Outport
  wires:
  Transfer Fcn/1 -> Product/2
  mass/1 -> Product/1
  flight_path_com/1 -> Sin/1
  Sin/1 -> Subtract/1, Product2/3
  flight_path/1 -> Sin1/1
  Sin1/1 -> Subtract/2
  Subtract/1 -> Product1/2
  groundspeed_com/1 -> Product2/2, Product1/1
  Product1/1 -> Transfer Fcn/1
  Product/1 -> Transfer Fcn1/1, MATLAB Function/3(L_c), To Workspace2/1
  groundspeed/1 -> Square/1
  Square/1 -> Gain/1
  Gain/1 -> MATLAB Function/4(L_max), Saturation Dynamic/1, To Workspace3/1  "lift_max"
  airspeed/1 -> MATLAB Function/2(airspeed)
  Transfer Fcn1/1 -> Saturation Dynamic/2
  Saturation Dynamic/1 -> MATLAB Function/1(L), lift/1, To Workspace/1
  Zero/1 -> Saturation Dynamic/3
  Clock/1 -> Product2/1
  Product2/1 -> Sum/1
  Constant/1 -> Sum/2
  Sum/1 -> To Workspace7/1, Scope/1
  MATLAB Function/1(alpha_c) -> Radians to Degrees/1
  Radians to Degrees/1 -> To Workspace4/1
  MATLAB Function/2(alpha) -> Radians to Degrees1/1
  Radians to Degrees1/1 -> To Workspace1/1
  MATLAB Function/3(alpha_max) -> Radians to Degrees2/1
  Radians to Degrees2/1 -> To Workspace6/1

== system OswaldE_Proj2_Sim/Simplified Simulation/Guidance & Control System/Thrust Guidance Law & Controller Dynamics ==
  mass : Inport
  groundspeed_com : Inport  Port=2
  groundspeed : Inport  Port=3
  Product : Product
  Saturation : Saturate  UpperLimit=T_max  LowerLimit=0
  Subtract : Sum  Inputs=+-
  To Workspace : ToWorkspace  VariableName=thrust
  To Workspace1 : ToWorkspace  VariableName=thrust_com
  Transfer Fcn : TransferFcn  Numerator=[KT_p KT_i]  Denominator=[1 0]
  Transfer Fcn1 : TransferFcn  Numerator=[0 omega_t]  Denominator=[1 omega_t]
  thrust : Outport
  wires:
  Transfer Fcn/1 -> Product/2
  mass/1 -> Product/1
  groundspeed_com/1 -> Subtract/1
  groundspeed/1 -> Subtract/2
  Subtract/1 -> Transfer Fcn/1
  Product/1 -> To Workspace1/1, Transfer Fcn1/1
  Transfer Fcn1/1 -> Saturation/1
  Saturation/1 -> thrust/1, To Workspace/1

== system OswaldE_Proj2_Sim/Simplified Simulation/Vehicle Dynamics/Flight Path Rate Equation ==
  groundspeed : Inport
  mass : Inport  Port=2
  "lift " : Inport  Port=3
  bank : Inport  Port=4
  Integrator : Integrator  InitialCondition=gamma_0
  MATLAB Function : MATLAB Function  TreatAsAtomicUnit=on
  flight path : Outport
  wires:
  groundspeed/1 -> MATLAB Function/2(v)
  mass/1 -> MATLAB Function/5(m)
  "lift "/1 -> MATLAB Function/1(L)
  bank/1 -> MATLAB Function/3(mu)
  MATLAB Function/1(gamma_der) -> Integrator/1
  Integrator/1 -> MATLAB Function/4(gamma), flight path/1

== system OswaldE_Proj2_Sim/Simplified Simulation/Vehicle Dynamics/Groundspeed Rate Equation ==
  mass : Inport
  lift : Inport  Port=2
  thrust : Inport  Port=3
  flight path : Inport  Port=4
  airspeed : Inport  Port=5
  Integrator : Integrator  InitialCondition=v_bn_0
  MATLAB Function : MATLAB Function  TreatAsAtomicUnit=on
  MATLAB Function1 : MATLAB Function  TreatAsAtomicUnit=on
  To Workspace3 : ToWorkspace  VariableName=drag
  rho : Constant  Value=2.3769*10^-3
  groundspeed : Outport
  wires:
  airspeed/1 -> MATLAB Function/2(V_mag)
  lift/1 -> MATLAB Function/3(L)
  Integrator/1 -> groundspeed/1
  rho/1 -> MATLAB Function/1(rho)
  MATLAB Function/1(D) -> To Workspace3/1, MATLAB Function1/1(D)
  thrust/1 -> MATLAB Function1/2(T)
  mass/1 -> MATLAB Function1/4(m)
  flight path/1 -> MATLAB Function1/3(gamma)
  MATLAB Function1/1(v_der) -> Integrator/1

== system OswaldE_Proj2_Sim/Simplified Simulation/Vehicle Dynamics/Heading Rate Equation ==
  flight path : Inport
  groundspeed : Inport  Port=2
  mass : Inport  Port=3
  "lift " : Inport  Port=4
  bank : Inport  Port=5
  Integrator : Integrator  InitialCondition=sigma_0
  MATLAB Function : MATLAB Function  TreatAsAtomicUnit=on
  heading : Outport
  wires:
  "lift "/1 -> MATLAB Function/1(L)
  bank/1 -> MATLAB Function/3(bank)
  mass/1 -> MATLAB Function/2(m)
  groundspeed/1 -> MATLAB Function/4(v)
  flight path/1 -> MATLAB Function/5(gamma)
  MATLAB Function/1(head_der) -> Integrator/1
  Integrator/1 -> heading/1

== system OswaldE_Proj2_Sim/Simplified Simulation/Vehicle Dynamics/Inertial Position and Airspeed ==
  groundspeed : Inport
  "flight path " : Inport  Port=2
  heading : Inport  Port=3
  Integrator : Integrator  InitialCondition=lat_0
  Integrator1 : Integrator  InitialCondition=long_0
  Integrator2 : Integrator  InitialCondition=h_0
  MATLAB Function : MATLAB Function  TreatAsAtomicUnit=on
  latitude : Outport
  longitude : Outport  Port=2
  altitude : Outport  Port=3
  airspeed : Outport  Port=4
  wires:
  MATLAB Function/1(lat_der) -> Integrator/1
  Integrator/1 -> MATLAB Function/4(lat), latitude/1
  MATLAB Function/2(long_der) -> Integrator1/1
  Integrator1/1 -> longitude/1
  "flight path "/1 -> MATLAB Function/3(gamma)
  heading/1 -> MATLAB Function/2(head)
  groundspeed/1 -> MATLAB Function/1(v)
  MATLAB Function/3(h_der) -> Integrator2/1
  Integrator2/1 -> MATLAB Function/5(h), altitude/1
  MATLAB Function/4(windspeed) -> airspeed/1

== system OswaldE_Proj2_Sim/Simplified Simulation/Vehicle Dynamics/Mass Rate Equation ==
  thrust : Inport
  Gain : Gain  Gain=-K_f
  Gain1 : Gain  Gain=g0
  Integrator : Integrator  InitialCondition=200000/g0
  To Workspace2 : ToWorkspace  VariableName=weight
  "mass " : Outport
  wires:
  thrust/1 -> Gain/1
  Gain1/1 -> To Workspace2/1
  Gain/1 -> Integrator/1
  Integrator/1 -> Gain1/1, "mass "/1

== matlab function OswaldE_Proj2_Sim/Complex Simulation/Planning System1/Command System ==
  data: latitude input; groundspeed_com output; longitude input; altitude input; flight_path_com output; heading_com output
function [groundspeed_com, flight_path_com, heading_com] = ...
    command_trajectory(latitude, longitude, altitude)
% Define the commanded velocity, flight path and heading

FPS2MPH = 3600/5280;
DEG2RAD = pi/180;

groundspeed_com = 450/FPS2MPH;          % fps
flight_path_com = 5*DEG2RAD;    % rad
heading_com = 15*DEG2RAD;          % rad

end

== matlab function OswaldE_Proj2_Sim/Complex Simulation/Vehicle Dynamics1/Flight Path Rate Equation/MATLAB Function ==
  data: L input; gamma_der output; v input; mu input; gamma input; m input; g input; F_app2 input; F_app3 input; alpha input; T input
function gamma_der = fcn(L,v,mu,gamma,m, g, F_app2, F_app3, alpha, T)

gamma_der = 1/v *((L+T*sin(alpha))/m * cos(mu) - g*cos(gamma) - (F_app2*sin(mu) + F_app3*cos(mu)));

== matlab function OswaldE_Proj2_Sim/Complex Simulation/Vehicle Dynamics1/Groundspeed Rate Equation/MATLAB Function ==
  data: rho input; D output; V_mag input; L input
function D = fcn(rho, V_mag, L)
S_w = 1745;
C_D_0 = .0183;
AR_w = 10.1;
e_eff = .613;
D = 1/2 * rho * S_w * C_D_0 * V_mag^2 + (2/(rho*S_w*pi*AR_w*e_eff)) * L^2/V_mag^2;

== matlab function OswaldE_Proj2_Sim/Complex Simulation/Vehicle Dynamics1/Groundspeed Rate Equation/MATLAB Function1 ==
  data: D input; v_der output; T input; gamma input; g input; F_app1 input; m input; alpha input
function v_der = fcn(D,T,gamma,g, F_app1, m, alpha)

v_der = (T*cos(alpha)-D)/m - g * sin(gamma) + F_app1;

== matlab function OswaldE_Proj2_Sim/Complex Simulation/Vehicle Dynamics1/Heading Rate Equation/MATLAB Function ==
  data: L input; head_der output; m input; bank input; v input; gamma input; T input; alpha input; F_app2 input; F_app3 input
function head_der = fcn(L,m,bank,v,gamma, T, alpha,F_app2,F_app3)
head_der = 1/(v*cos(gamma)) * ((L+T*sin(alpha))/m * sin(bank) + (F_app2*sin(bank) - F_app3*sin(bank)));

== matlab function OswaldE_Proj2_Sim/Complex Simulation/Vehicle Dynamics1/Inertial Position and Airspeed/MATLAB Function ==
  data: v input; lat_der output; head input; gamma input; lat input; long_der output; h_der output; windspeed output; h input
function [lat_der,long_der,h_der, windspeed] = fcn(v, head, gamma, lat,h)
Re = 6371000;
v_wn_n = [40;40;0];
lat_der = (v*cos(gamma)*cos(head))/(Re+h);
long_der = v*cos(gamma)*sin(head)/((Re+h)*cos(lat));
h_der = v*sin(gamma);
velocity = [v*cos(gamma)*cos(head);v*cos(gamma)*sin(head);v*sin(gamma)] - v_wn_n;
windspeed = norm(velocity);

== matlab function OswaldE_Proj2_Sim/Simplified Simulation/Planning System/Command System ==
  data: latitude input; groundspeed_com output; longitude input; altitude input; flight_path_com output; heading_com output
function [groundspeed_com, flight_path_com, heading_com] = ...
    command_trajectory(latitude, longitude, altitude)
% Define the commanded velocity, flight path and heading

FPS2MPH = 3600/5280;
DEG2RAD = pi/180;

groundspeed_com = 450/FPS2MPH;          % fps
flight_path_com = 5*DEG2RAD;    % rad
heading_com = 15*DEG2RAD;          % rad

end

== matlab function OswaldE_Proj2_Sim/Complex Simulation/Vehicle Dynamics1/Density and Grav. Accel Calc/MATLAB Function ==
  data: h input; rho output; lat input; g output
function [rho, g] = fcn(h, lat)
g0 = 32.17;
Re = 6371000;

if h > 0 && h < 36089
    rho = 6.6277*10^-15 * (518.69 - (3.5662*10^-3)*h)^4.256;
elseif h < 65617
    rho = 1.4939*10^-6 * (2678.4) *exp(-4.8063*10^-5*h);
else
    rho = 2.2099*10^87 * (389.99+(5.4864*10^-4)*(h-65617))^-35.164;
end

g = g0 * lat * (Re/(Re+h))^2;

== matlab function OswaldE_Proj2_Sim/Complex Simulation/Vehicle Dynamics1/pqr/MATLAB Function ==
  data: lat input; long_der input; lat_der input; gamma input; r_ni output; bank input; head input; r_ei output; q_ni output; q_ei output
function [r_ni, r_ei, q_ni, q_ei] = fcn(lat, long_der, lat_der, gamma,bank,head)
omega_e = 7.292*10^-5;

C_wn = [cos(gamma)*cos(head), cos(gamma)*sin(head), -sin(gamma);...
       sin(bank)*sin(gamma)*cos(head) - cos(bank)*sin(head), sin(bank)*sin(gamma)*sin(head) + cos(bank)*cos(head), sin(bank)*cos(gamma);...
       cos(bank)*sin(gamma)*cos(head) + sin(bank)*sin(head), cos(bank)*sin(gamma)*sin(head) - sin(bank)*cos(head), cos(bank)*cos(gamma)];

mat1 = C_wn * [(omega_e + long_der)*cos(lat); -lat_der; -(omega_e + long_der)*sin(lat)];

mat2 = C_wn * [omega_e*cos(lat);0;-omega_e*sin(lat)];

r_ni = mat1(3);
r_ei = mat2(3);
q_ni = mat1(2);
q_ei = mat2(2);

== matlab function OswaldE_Proj2_Sim/Complex Simulation/Vehicle Dynamics1/F_app/MATLAB Function ==
  data: long input; gamma input; h input; v input; Fapp_1 output; head input; r_ni input; r_ei input; q_ei input; q_ni input; bank input; Fapp_2 output; Fapp_3 output
function [Fapp_1, Fapp_2, Fapp_3] = fcn(long, gamma, h, v, head, r_ni, r_ei, q_ei, q_ni, bank)

Re = 6371000;
omega_e = 7.292*10^-5;
Fapp_1 = -omega_e^2*(Re+h)*cos(long)*(sin(long)*cos(gamma)*cos(head)-cos(long)*sin(gamma));
Fapp_2 = -r_ni*v - r_ei*v -omega_e^2*(Re+h)*cos(long)*(sin(long)*(sin(bank)*sin(gamma)*cos(head) - cos(bank)*sin(head)) + cos(long)*sin(bank)*cos(gamma));
Fapp_3 = q_ni*v +q_ei*v -omega_e^2*(Re+h)*cos(long)*(sin(long)*(cos(bank)*sin(gamma)*cos(head) + sin(bank)*sin(head)) + cos(long)*cos(bank)*cos(gamma));

== matlab function OswaldE_Proj2_Sim/Simplified Simulation/Vehicle Dynamics/Groundspeed Rate Equation/MATLAB Function ==
  data: rho input; D output; V_mag input; L input
function D = fcn(rho, V_mag, L)
S_w = 1745;
C_D_0 = .0183;
AR_w = 10.1;
e_eff = .613;
D = 1/2 * rho * S_w * C_D_0 * V_mag^2 + (2/(rho*S_w*pi*AR_w*e_eff)) * L^2/V_mag^2;

== matlab function OswaldE_Proj2_Sim/Simplified Simulation/Vehicle Dynamics/Groundspeed Rate Equation/MATLAB Function1 ==
  data: D input; v_der output; T input; gamma input; m input
function v_der = fcn(D,T,gamma,m)
g0 = 32.17;
v_der = (T-D)/m - g0 * sin(gamma);

== matlab function OswaldE_Proj2_Sim/Simplified Simulation/Vehicle Dynamics/Flight Path Rate Equation/MATLAB Function ==
  data: L input; gamma_der output; v input; mu input; gamma input; m input
function gamma_der = fcn(L,v,mu,gamma,m)
g0 = 32.17;
gamma_der = 1/v *(L/m * cos(mu) - g0*cos(gamma));

== matlab function OswaldE_Proj2_Sim/Simplified Simulation/Vehicle Dynamics/Heading Rate Equation/MATLAB Function ==
  data: L input; head_der output; m input; bank input; v input; gamma input
function head_der = fcn(L,m,bank,v,gamma)
head_der = 1/(v*cos(gamma)) * ((L)/m * sin(bank));

== matlab function OswaldE_Proj2_Sim/Simplified Simulation/Vehicle Dynamics/Inertial Position and Airspeed/MATLAB Function ==
  data: v input; lat_der output; head input; gamma input; lat input; long_der output; h_der output; windspeed output; h input
function [lat_der,long_der,h_der, windspeed] = fcn(v, head, gamma, lat,h)
Re = 6371000;
v_wn_n = [40;40;0];
lat_der = (v*cos(gamma)*cos(head))/(Re+h);
long_der = v*cos(gamma)*sin(head)/((Re+h)*cos(lat));
h_der = v*sin(gamma);
velocity = [v*cos(gamma)*cos(head);v*cos(gamma)*sin(head);v*sin(gamma)] - v_wn_n;
windspeed = norm(velocity);

== matlab function OswaldE_Proj2_Sim/Simplified Simulation/Guidance & Control System/Lift Guidance Law & Controller Dynamics/MATLAB Function ==
  data: L input; alpha_c output; airspeed input; L_c input; alpha output; L_max input; alpha_max output
function [alpha_c,alpha, alpha_max] = fcn(L,airspeed,L_c, L_max)
rho = 2.3769 * 10^-3;
S_w = 1745;
C_L_alpha = .092 * 180/pi;
alpha_0 = -.05 * pi/180;
alpha = 2/(rho * S_w * C_L_alpha) * L/airspeed^2 + alpha_0;
alpha_c = 2/(rho * S_w * C_L_alpha) * L_c/airspeed^2 + alpha_0;
alpha_max = 2/(rho * S_w * C_L_alpha) * L_max/airspeed^2 + alpha_0;

== matlab function OswaldE_Proj2_Sim/Complex Simulation/Guidance & Control System1/Lift Guidance Law & Controller Dynamics/MATLAB Function ==
  data: L input; alpha_c output; airspeed input; L_c input; alpha output; L_max input; alpha_max output; rho input
function [alpha_c,alpha, alpha_max] = fcn(L,airspeed,L_c, L_max, rho)
S_w = 1745;
C_L_alpha = .092 * 180/pi;
alpha_0 = -.05 * pi/180;
alpha = 2/(rho * S_w * C_L_alpha) * L/airspeed^2 + alpha_0;
alpha_c = 2/(rho * S_w * C_L_alpha) * L_c/airspeed^2 + alpha_0;
alpha_max = 2/(rho * S_w * C_L_alpha) * L_max/airspeed^2 + alpha_0;
